simulink model "Yaw_Discrete_Servo_OutputFeedback"  (R2018b)
settings: Solver=VariableStepAuto  StartTime=0.0  StopTime=30  RelTol=1e-3
undefined symbols (not defined in the file): Gyawd_A_obs, Gyawd_B_obs, Gyawd_C_obs, K0_yaw, K_yaw, KGe_yaw, t_samp
libraries: simulink x1
settings Model: Creator=User  LastModifiedBy=User

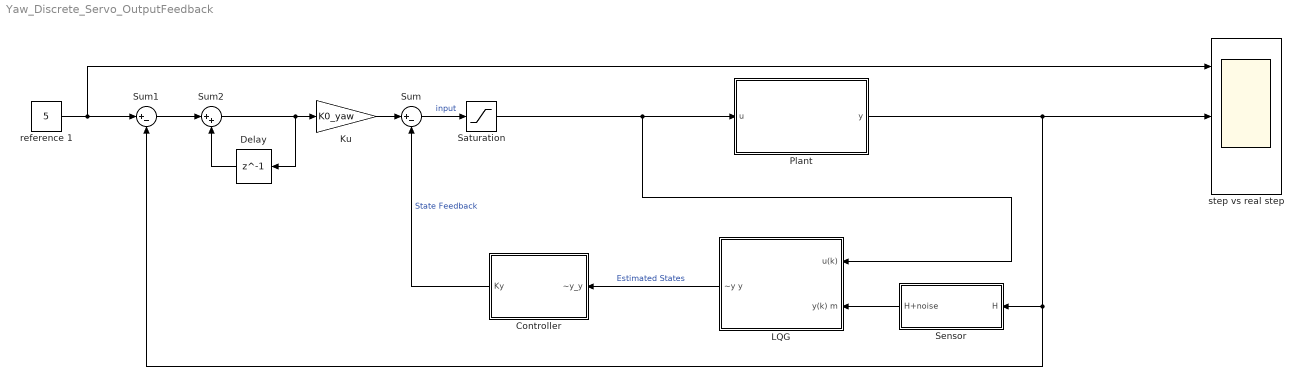
== system Yaw_Discrete_Servo_OutputFeedback ==
  "Controller " : Subsystem
  Delay : Delay  DelayLength=1  InitialCondition=0
  Ku : Gain  Gain=K0_yaw
  "LQG " : Subsystem
  Plant : Subsystem
  Saturation : Saturate  UpperLimit=1.2  LowerLimit=-1.2
  Sensor : Subsystem
  Sum : Sum  Inputs=|+-
  Sum1 : Sum  Inputs=|+-
  Sum2 : Sum  Inputs=|++
  reference 1 : Constant  Value=5
  "step vs real step " : Scope  NumInputPorts=3
  wires:
  reference 1/1 -> Sum1/1, "step vs real step "/1
  "Controller "/1(Ky) -> Sum/2  "State Feedback"
  "LQG "/1("~y y ") -> "Controller "/1(~y_y)  "Estimated States"
  Saturation/1 -> "LQG "/1(u(k)), Plant/1("u ")
  Sum/1 -> Saturation/1  "input"
  Sensor/1(H+noise) -> "LQG "/2(y(k) m)
  Plant/1("y ") -> Sum1/2, Sensor/1(H), "step vs real step "/2
  Delay/1 -> Sum2/2
  Sum1/1 -> Sum2/1
  Sum2/1 -> Delay/1, Ku/1
  Ku/1 -> Sum/1

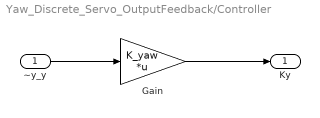
== system Yaw_Discrete_Servo_OutputFeedback/Controller  ==
  ~y_y : Inport
  Gain : Gain  Gain=K_yaw  Multiplication=Matrix(K*u) (u vector)
  Ky : Outport
  wires:
  ~y_y/1 -> Gain/1
  Gain/1 -> Ky/1

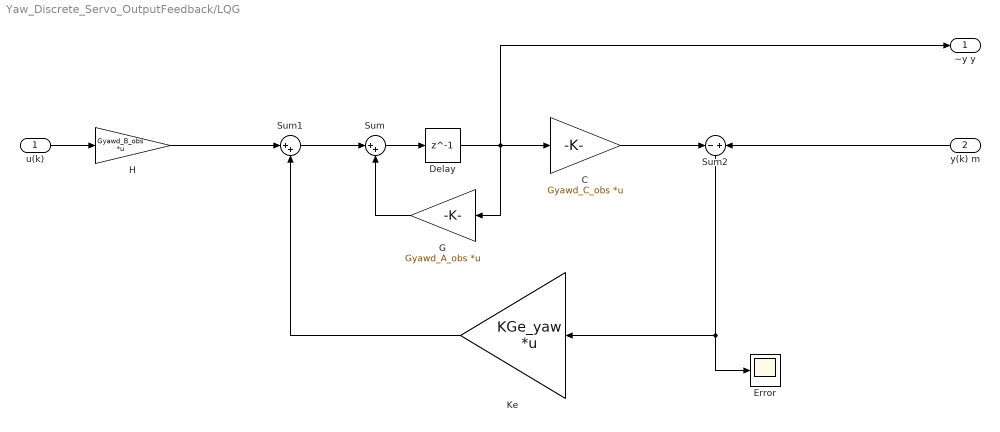
== system Yaw_Discrete_Servo_OutputFeedback/LQG  ==
  u(k) : Inport
  y(k) m : Inport  Port=2
  C : Gain  Gain=Gyawd_C_obs  Multiplication=Matrix(K*u)
  Delay : Delay  DelayLength=1  InitialCondition=0  SampleTime=t_samp
  Error : Scope
  G : Gain  Gain=Gyawd_A_obs  Multiplication=Matrix(K*u)
  H : Gain  Gain=Gyawd_B_obs  Multiplication=Matrix(K*u)
  Ke : Gain  Gain=KGe_yaw  Multiplication=Matrix(K*u)
  Sum : Sum  Inputs=|++
  Sum1 : Sum  Inputs=|++
  Sum2 : Sum  Inputs=-+
  "~y y " : Outport
  wires:
  C/1 -> Sum2/1
  y(k) m/1 -> Sum2/2
  H/1 -> Sum1/1
  Sum/1 -> Delay/1
  u(k)/1 -> H/1
  G/1 -> Sum/2
  Sum2/1 -> Error/1, Ke/1
  Sum1/1 -> Sum/1
  Ke/1 -> Sum1/2
  Delay/1 -> "~y y "/1, G/1, C/1

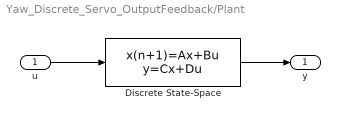
== system Yaw_Discrete_Servo_OutputFeedback/Plant ==
  "u " : Inport
  Discrete State-Space : DiscreteStateSpace  A=Gyawd_A_obs  B=Gyawd_B_obs  C=Gyawd_C_obs  D=0  SampleTime=t_samp
  "y " : Outport
  wires:
  "u "/1 -> Discrete State-Space/1
  Discrete State-Space/1 -> "y "/1

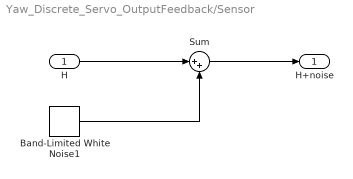
== system Yaw_Discrete_Servo_OutputFeedback/Sensor ==
  H : Inport
  Band-Limited White Noise1 : simulink/Sources/Band-Limited White Noise  Cov=.00001  Ts=0.1  seed=[124553]
  Sum : Sum  Inputs=|++
  H+noise : Outport
  wires:
  Sum/1 -> H+noise/1
  H/1 -> Sum/1
  Band-Limited White Noise1/1 -> Sum/2
